simulink model "mass"  (Simulink 7.6)
settings: Solver=ode4  StartTime=0.0  StopTime=20  FixedStep=0.01  RelTol=1e-3
values from neighbouring files (symbols this model uses):
  m = 10    [DrawingTest.m]    (also in MasterP_2DMassData_BEST.m = 100; MasterP_2DMassData_MAIN.m; MasterP_2DMassData_TEST.m = 100; MasterP_4DInvPendData_BEST.m)
undefined symbols (not defined in the file or in its folder): SU
libraries: simulink x1
settings Model: Creator=Mohsen  LastModifiedBy=Mohsen

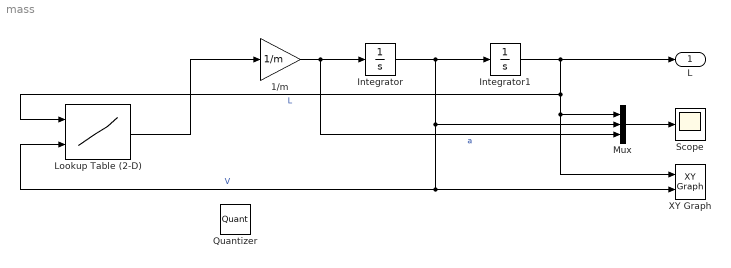
== system mass ==
  1/m : Gain  Gain=1/m
  Integrator : Integrator  InitialCondition=6
  Integrator1 : Integrator  InitialCondition=3
  Lookup Table (2-D) : Lookup2D  RowIndex=[-4:4]  ColumnIndex=[-8:2:8]  Table=SU
  Mux : Mux  Inputs=3
  Quantizer : Quantizer  QuantizationInterval=1
  Scope : Scope
      settings: TimeRange=20  YMin=-20  YMax=10  SaveName=states  DataFormat=Array
  XY Graph : simulink/Sinks/XY Graph  SystemSampleTime=-1  xmin=-5  xmax=5  ymin=-10  ymax=10  st=-1
  L : Outport
  wires:
  1/m/1 -> Integrator/1, Mux/3  "a"
  Integrator/1 -> Integrator1/1, Mux/2, XY Graph/2, Lookup Table (2-D)/2  "V"
  Integrator1/1 -> L/1, Mux/1, XY Graph/1, Lookup Table (2-D)/1  "L"
  Mux/1 -> Scope/1
  Lookup Table (2-D)/1 -> 1/m/1
